simulink subsystem "Sensor_Voltaje"  (R2023b)
settings: Solver=VariableStepAuto  StartTime=0.0  StopTime=10.0  RelTol=1e-3
libraries: arduinolib x1
settings Model: Creator=Manuel  LastModifiedBy=Manuel

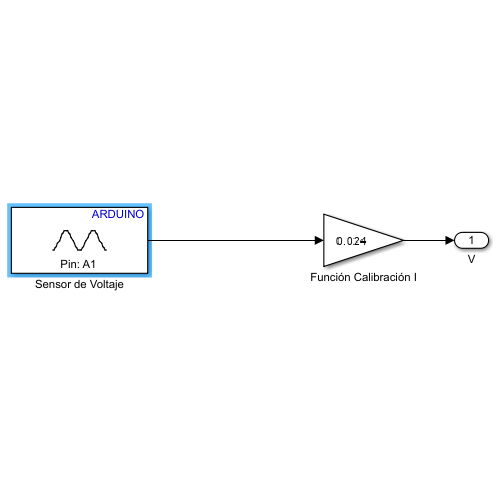
[thumbnail: Simulink's stored preview of the top-level diagram]
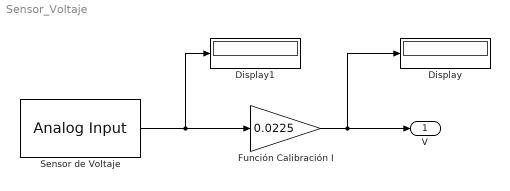
== system Sensor_Voltaje ==
  Display : Display
  Display1 : Display
  Función Calibración I : Gain  Gain=0.0225
  Sensor de Voltaje : arduinolib/Analog Input  pinNumber=1  ReadResultsOnly=off  ConversionTriggerSource=Software  ExternalTriggerType=uint32( 0 )  OutputDataType=uint16  EnableConversionCompleteNotify=off  EnableOuputStatus=off  SampleTime=-1  blockPlatform=arduino
  V : Outport
  wires:
  Función Calibración I/1 -> V/1, Display/1
  Sensor de Voltaje/1 -> Función Calibración I/1, Display1/1
